simulink model "ej8"  (R2023a)
settings: Solver=VariableStepAuto  StartTime=0.0  StopTime=100  MaxStep=0.01  RelTol=1e-3
settings Model: Creator=santi  LastModifiedBy=santi

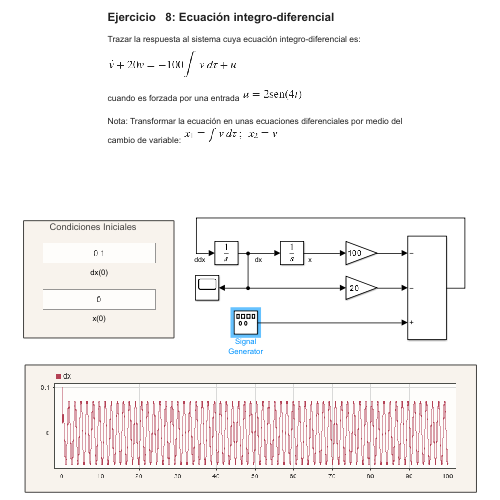
[thumbnail: Simulink's stored preview of the top-level diagram]
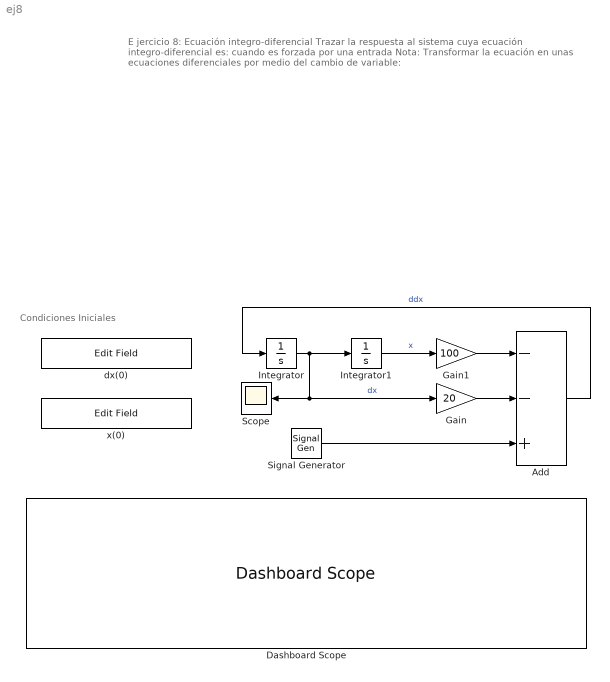
== system ej8 ==
  note: Condiciones Iniciales
  note: E jercicio 8: Ecuación integro-diferencial
      | Trazar la respuesta al sistema cuya ecuación integro-diferencial es:
      |
      | cuando es forzada por una entrada
      | Nota: Transformar la ecuación en unas ecuaciones diferenciales por medio del cambio de variable:
  Add : Sum  Inputs=--+
  Dashboard Scope : DashboardScope  ShowInitialText=off  NormalizeYAxis=on
  Gain : Gain  Gain=20
  Gain1 : Gain  Gain=100
  Integrator : Integrator  InitialCondition=0.1
  Integrator1 : Integrator
  Scope : Scope
  Signal Generator : SignalGenerator  Amplitude=2  Frequency=4  Units=rad/sec
  dx(0) : EditField  LabelPosition=Hide  ShowInitialText=on  Alignment=Center
  x(0) : EditField  LabelPosition=Hide  ShowInitialText=on  Alignment=Center
  wires:
  Integrator/1 -> Scope/1, Gain/1, Integrator1/1  "dx"
  Integrator1/1 -> Gain1/1  "x"
  Add/1 -> Integrator/1  "ddx"
  Gain1/1 -> Add/1
  Gain/1 -> Add/2
  Signal Generator/1 -> Add/3
